simulink model "model"  (R2016a)
settings: Solver=VariableStepAuto  StartTime=0.0  StopTime=10.0  RelTol=1e-3
settings Model: Creator=SPDKH  LastModifiedBy=SPDKH

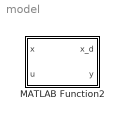
== system model ==
  MATLAB Function2 : MATLAB Function  TreatAsAtomicUnit=on

== matlab function model/MATLAB Function2 ==
  data: x input; u input; x_d output; y output
function [x_d,y]= fcn(x,u)

A = [-6.0476 -5.2856 -0.2380;1.0000 0 0; 0 1.0000 0];
B =[1 0 0]';
C =[0 0 2.4767];

x_d = A*x +B*u;
y = C*x;
